simulink model "Quarter_Car_Model"  (R2020b)
settings: Solver=VariableStepAuto  StartTime=0.0  StopTime=10.0  RelTol=1e-3
model workspace (MAT data in the model file):
  b = 1
  ks = 1
  kw = 1
settings Model: Creator=oplat  LastModifiedBy=oplat

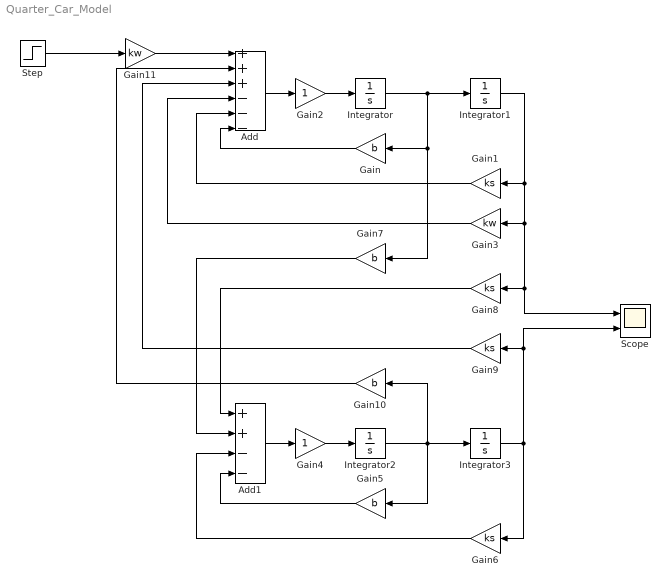
== system Quarter_Car_Model ==
  Add : Sum  Inputs=+++---
  Add1 : Sum  Inputs=++--
  Gain{,5,7,10} (4 alike) : Gain  Gain=b
  Gain{1,6,8..9} (4 alike) : Gain  Gain=ks
  Gain11 : Gain  Gain=kw
  Gain2 : Gain
  Gain3 : Gain  Gain=kw
  Gain4 : Gain
  Integrator{,1..3} (4 alike) : Integrator
  Scope : Scope  NumInputPorts=2
  Step : Step  SampleTime=0
  wires:
  Integrator/1 -> Gain7/1, Gain/1, Integrator1/1
  Integrator1/1 -> Scope/1, Gain8/1, Gain3/1, Gain1/1
  Gain/1 -> Add/6
  Gain1/1 -> Add/5
  Add/1 -> Gain2/1
  Gain2/1 -> Integrator/1
  Gain3/1 -> Add/4
  Add1/1 -> Gain4/1
  Gain4/1 -> Integrator2/1
  Integrator2/1 -> Gain10/1, Gain5/1, Integrator3/1
  Gain5/1 -> Add1/4
  Integrator3/1 -> Gain6/1, Gain9/1, Scope/2
  Gain6/1 -> Add1/3
  Gain8/1 -> Add1/1
  Gain7/1 -> Add1/2
  Gain9/1 -> Add/3
  Gain10/1 -> Add/2
  Step/1 -> Gain11/1
  Gain11/1 -> Add/1
